simulink model "lab7"  (R2013a)
settings: Solver=ode23tb  StartTime=0.0  StopTime=5  RelTol=1e-3
libraries: powerlib x23, powerlib_meascontrol x2
settings Model: Creator=Erika  LastModifiedBy=Erika

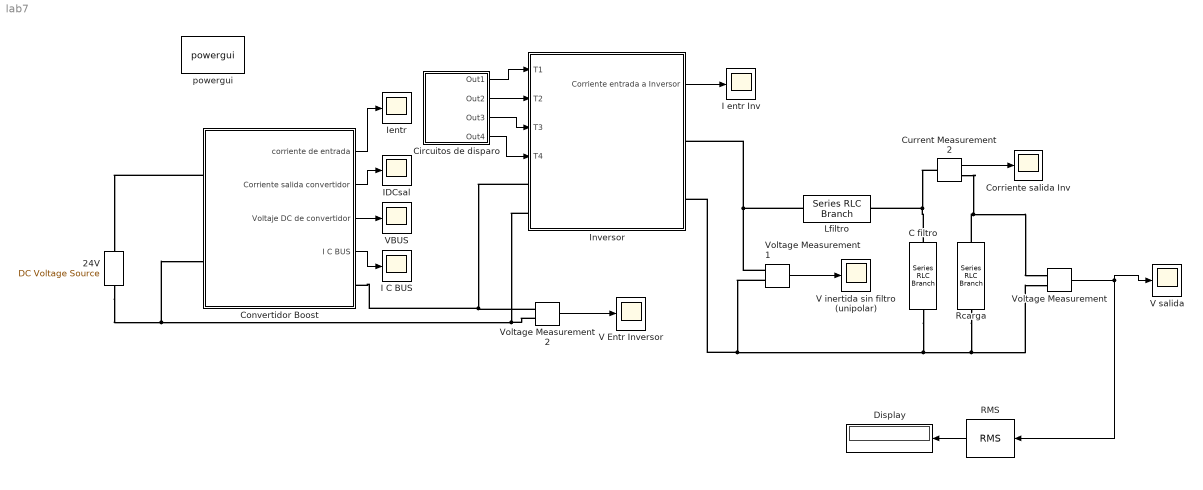
== system lab7 ==
  24V : powerlib/Electrical Sources/DC Voltage Source  Amplitude=24  Measurements=None
  C filtro : powerlib/Elements/Series RLC Branch  LConnTagsString=__new0  RConnTagsString=__new0  BranchType=C  Resistance=1  Inductance=1e-3  SetiL0=off  InitialCurrent=0  Capacitance=104.24e-9  Setx0=off  InitialVoltage=0  Measurements=None
  Circuitos de disparo : Subsystem
  Convertidor Boost : Subsystem
  Corriente salida Inv : Scope
      settings: SaveName=ScopeData5  MaxDataPoints=500000
  Current Measurement2 : powerlib/Measurements/Current Measurement  PhasorSimulation=off  OutputType=Complex  PSBequivalent=0
  Display : Display
  I C BUS : Scope
      settings: TimeRange=0.004770167640737899  YMin=198.7058285790732  YMax=199.7217120353623  SaveName=ScopeData7  MaxDataPoints=5000000
  I entr Inv : Scope
      settings: SaveName=ScopeData4  MaxDataPoints=500000
  IDCsal : Scope
      settings: SaveName=ScopeData3  MaxDataPoints=500000
  Ientr : Scope
      settings: SaveName=ScopeData2  MaxDataPoints=500000
  Inversor : Subsystem
  Lfiltro : powerlib/Elements/Series RLC Branch  LConnTagsString=__new0  RConnTagsString=__new0  BranchType=L  Resistance=1  Inductance=0.3  SetiL0=off  InitialCurrent=0  Capacitance=1e-6  Setx0=off  InitialVoltage=0  Measurements=None
  RMS : powerlib_meascontrol/Measurements/RMS  TrueRMS=on  Freq=60  RMSInit=120  Ts=0
  Rcarga : powerlib/Elements/Series RLC Branch  LConnTagsString=__new0  RConnTagsString=__new0  BranchType=RL  Resistance=720  Inductance=1.1836  SetiL0=off  InitialCurrent=0  Capacitance=1e-6  Setx0=off  InitialVoltage=0  Measurements=None
  V Entr Inversor : Scope
      settings: SaveName=ScopeData6  MaxDataPoints=500000
  V inertida sin filtro (unipolar) : Scope
      settings: SaveName=ScopeData8  MaxDataPoints=500000
  V salida : Scope
      settings: MaxDataPoints=500000
  VBUS : Scope
      settings: TimeRange=0.004770167640737899  YMin=198.7058285790732  YMax=199.7217120353623  MaxDataPoints=5000000
  Voltage Measurement : powerlib/Measurements/Voltage Measurement  PhasorSimulation=off  OutputType=Complex  PSBequivalent=0
  Voltage Measurement1 : powerlib/Measurements/Voltage Measurement  PhasorSimulation=off  OutputType=Complex  PSBequivalent=0
  Voltage Measurement2 : powerlib/Measurements/Voltage Measurement  PhasorSimulation=off  OutputType=Complex  PSBequivalent=0
  powergui : powerlib/powergui  Priority=1  SimulationMode=Discrete  SolverType=Tustin  SampleTime=2e-6  frequency=60  SPID=off  DisableSnubberDevices=off  DisableRonSwitches=off  DisableVfSwitches=off  SwTol=0  Interpol=off  DisplayEquations=off  frequencyindice=0  Pbase=100e6  ErrMax=1e-4  Iterations=50  UnitsV=kV  UnitsW=MW  FunctionMessages=off  echomessages=off  HookPort=off  EnableUseOfTLC=off  x0status=blocks  RestoreLinks=warning  ResistiveCurrentMeasurement=off  Frange=[0:2:500]  Ylog=off  Xlog=on  ShowGrid=off  save=off  variable=ZData  ZoomFFT=off  StartTime=0.0  cycles=1  DisplayStyle=1  fundamental=60  FreqAxis=off  MaxFrequency=1000  frequencyindicesteady=1  RmsSteady=1  display=off  Ts=0  methode=off
  wires:
  Voltage Measurement/1 -> V salida/1, RMS/1
  RMS/1 -> Display/1
  Current Measurement2/1 -> Corriente salida Inv/1
  Voltage Measurement2/1 -> V Entr Inversor/1
  Convertidor Boost/1(corriente de entrada) -> Ientr/1
  Convertidor Boost/2(Corriente salida convertidor) -> IDCsal/1
  Convertidor Boost/3(Voltaje DC de convertidor) -> VBUS/1
  Inversor/1(Corriente entrada a Inversor) -> I entr Inv/1
  Voltage Measurement1/1 -> V inertida sin filtro (unipolar)/1
  Circuitos de disparo/1(Out1) -> Inversor/1(T1)
  Circuitos de disparo/2(Out2) -> Inversor/2(T2)
  Circuitos de disparo/3(Out3) -> Inversor/3(T3)
  Circuitos de disparo/4(Out4) -> Inversor/4(T4)
  Convertidor Boost/4(I C BUS) -> I C BUS/1
  connections:
  C filtro/LConn1 -- Current Measurement2/LConn1 -- Lfiltro/RConn1
  Rcarga/LConn1 -- Current Measurement2/RConn1 -- Voltage Measurement/LConn1
  24V/LConn1 -- Inversor/LConn2 -- Voltage Measurement2/LConn2 -- Convertidor Boost/LConn2
  Voltage Measurement2/LConn1 -- Inversor/LConn1 -- Convertidor Boost/RConn1
  Convertidor Boost/LConn1 -- 24V/RConn1
  C filtro/RConn1 -- Voltage Measurement1/LConn2 -- Inversor/RConn2 -- Rcarga/RConn1 -- Voltage Measurement/LConn2
  Lfiltro/LConn1 -- Voltage Measurement1/LConn1 -- Inversor/RConn1

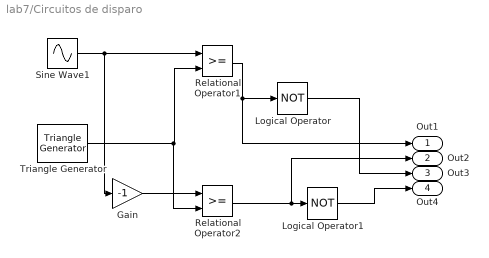
== system lab7/Circuitos de disparo ==
  Gain : Gain  Gain=-1
  Logical Operator : Logic  Operator=NOT  AllPortsSameDT=off  OutDataTypeStr=boolean
  Logical Operator1 : Logic  Operator=NOT  AllPortsSameDT=off  OutDataTypeStr=boolean
  Relational Operator1 : RelationalOperator  OutDataTypeStr=boolean
  Relational Operator2 : RelationalOperator  OutDataTypeStr=boolean
  Sine Wave1 : Sin  Amplitude=0.9  Frequency=2*pi*60  SampleTime=0
  Triangle Generator : powerlib_meascontrol/Pulse & Signal Generators/Triangle Generator  Freq=20000  Phase=90  Ts=0
  Out1 : Outport
  Out2 : Outport  Port=2
  Out3 : Outport  Port=3
  Out4 : Outport  Port=4
  wires:
  Logical Operator/1 -> Out3/1
  Logical Operator1/1 -> Out4/1
  Relational Operator1/1 -> Out1/1, Logical Operator/1
  Relational Operator2/1 -> Out2/1, Logical Operator1/1
  Gain/1 -> Relational Operator2/1
  Sine Wave1/1 -> Gain/1, Relational Operator1/1
  Triangle Generator/1 -> Relational Operator2/2, Relational Operator1/2

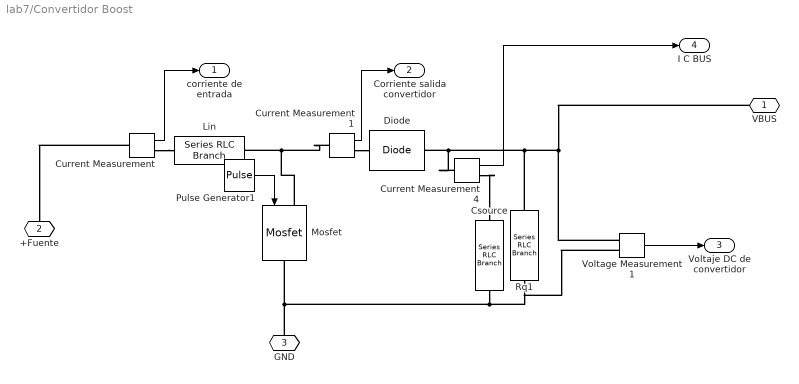
== system lab7/Convertidor Boost ==
  Csource : powerlib/Elements/Series RLC Branch  LConnTagsString=__new0  RConnTagsString=__new0  BranchType=C  Resistance=1  Inductance=1e-3  SetiL0=off  InitialCurrent=0  Capacitance=7.3142e-6  Setx0=off  InitialVoltage=0  Measurements=None
  Current Measurement : powerlib/Measurements/Current Measurement  PhasorSimulation=off  OutputType=Complex  PSBequivalent=0
  Current Measurement1 : powerlib/Measurements/Current Measurement  PhasorSimulation=off  OutputType=Complex  PSBequivalent=0
  Current Measurement4 : powerlib/Measurements/Current Measurement  PhasorSimulation=off  OutputType=Complex  PSBequivalent=0
  Diode : powerlib/Power Electronics/Diode  Ron=0.001  Lon=0  Vf=0.2  IC=0  UseSnubber=off  Rs=500  Cs=250e-9  Measurements=off
  Lin : powerlib/Elements/Series RLC Branch  LConnTagsString=__new0  RConnTagsString=__new0  BranchType=L  Resistance=1  Inductance=1.74658e-3  SetiL0=off  InitialCurrent=0  Capacitance=1e-6  Setx0=off  InitialVoltage=0  Measurements=None
  Mosfet : powerlib/Power Electronics/Mosfet  Ron=0.001  Lon=0  Rd=0.0001  Vfd=0  IC=0  Rs=1e6  Cs=inf  Measurements=off
  Pulse Generator1 : DiscretePulseGenerator  PulseType=Time based  Period=1/20000  PulseWidth=85
  Rq1 : powerlib/Elements/Series RLC Branch  LConnTagsString=__new0  RConnTagsString=__new0  BranchType=R  Resistance=494  Inductance=1e-3  SetiL0=off  InitialCurrent=0  Capacitance=1e-6  Setx0=off  InitialVoltage=0  Measurements=None
  Voltage Measurement1 : powerlib/Measurements/Voltage Measurement  PhasorSimulation=off  OutputType=Complex  PSBequivalent=0
  VBUS : PMIOPort  Port=1  Side=Right
  +Fuente : PMIOPort  Port=2  Side=Left
  GND : PMIOPort  Port=3  Side=Left
  corriente de entrada : Outport
  Corriente salida convertidor : Outport  Port=2
  Voltaje DC de convertidor : Outport  Port=3
  I C BUS : Outport  Port=4
  wires:
  Voltage Measurement1/1 -> Voltaje DC de convertidor/1
  Current Measurement4/1 -> I C BUS/1
  Current Measurement1/1 -> Corriente salida convertidor/1
  Pulse Generator1/1 -> Mosfet/1
  Current Measurement/1 -> corriente de entrada/1
  connections:
  Mosfet/LConn1 -- Current Measurement1/LConn1 -- Lin/RConn1
  Voltage Measurement1/LConn1 -- VBUS/RConn1 -- Rq1/LConn1 -- Current Measurement4/LConn1 -- Diode/RConn1
  Current Measurement4/RConn1 -- Csource/LConn1
  Current Measurement1/RConn1 -- Diode/LConn1
  Current Measurement/LConn1 -- +Fuente/RConn1
  Current Measurement/RConn1 -- Lin/LConn1
  GND/RConn1 -- Voltage Measurement1/LConn2 -- Rq1/RConn1 -- Csource/RConn1 -- Mosfet/RConn1

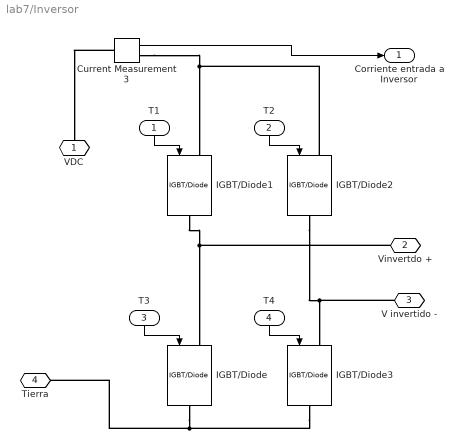
== system lab7/Inversor ==
  T1 : Inport
  T2 : Inport  Port=2
  T3 : Inport  Port=3
  T4 : Inport  Port=4
  Current Measurement3 : powerlib/Measurements/Current Measurement  PhasorSimulation=off  OutputType=Complex  PSBequivalent=0
  IGBT/Diode{,1..3} (4 alike) : powerlib/Power Electronics/IGBT//Diode  Ron=1e-3  Rs=1e5  Cs=inf  Measurements=off
  VDC : PMIOPort  Port=1  Side=Left
  Vinvertdo + : PMIOPort  Port=2  Side=Right
  V invertido - : PMIOPort  Port=3  Side=Right
  Tierra : PMIOPort  Port=4  Side=Left
  Corriente entrada a Inversor : Outport
  wires:
  Current Measurement3/1 -> Corriente entrada a Inversor/1
  T2/1 -> IGBT/Diode2/1
  T3/1 -> IGBT/Diode/1
  T1/1 -> IGBT/Diode1/1
  T4/1 -> IGBT/Diode3/1
  connections:
  IGBT/Diode2/RConn1 -- V invertido -/RConn1 -- IGBT/Diode3/LConn1
  IGBT/Diode1/RConn1 -- Vinvertdo +/RConn1 -- IGBT/Diode/LConn1
  IGBT/Diode2/LConn1 -- IGBT/Diode1/LConn1 -- Current Measurement3/RConn1
  Current Measurement3/LConn1 -- VDC/RConn1
  IGBT/Diode3/RConn1 -- Tierra/RConn1 -- IGBT/Diode/RConn1
